simulink model "Third_Order_Polynomial_Clean_Test_Harness"  (R2021b)
settings: Solver=FixedStepDiscrete  StartTime=0.0  StopTime=56  FixedStep=0.001  RelTol=1e-3
libraries: simulink_extras x2
settings Model: Creator=salva  LastModifiedBy=salva
settings DataIOCC: ReturnWorkspaceOutputsName=cubic_out
settings OptimizationCC: DefaultParameterBehavior=Inlined  EnhancedBackFolding=on  PassReuseOutputArgsAs=Individual arguments  ZeroExternalMemoryAtStartup=off  ZeroInternalMemoryAtStartup=off  OptimizeBlockOrder=speed  DifferentSizesBufferReuse=on  OptimizationCustomize=off  EfficientTunableParamExpr=on
settings DebuggingCC: ParameterTunabilityLossMsg=error
settings SFSimCC: MATLABDynamicMemAlloc=off
settings RTWCC: Description=Embedded Coder  SystemTargetFile=ert.tlc  TemplateMakefile=ert_default_tmf
settings CodeAppCC: ForceParamTrailComments=on  IgnoreCustomStorageClasses=off  OperatorAnnotations=on  SimulinkDataObjDesc=on  SFDataObjDesc=on  InsertBlockDesc=on
settings ERTTargetCC: TargetLangStandard=C99 (ISO)  GenerateSampleERTMain=on  InlinedParameterPlacement=NonHierarchical  ERTCustomFileTemplate=example_file_process.tlc

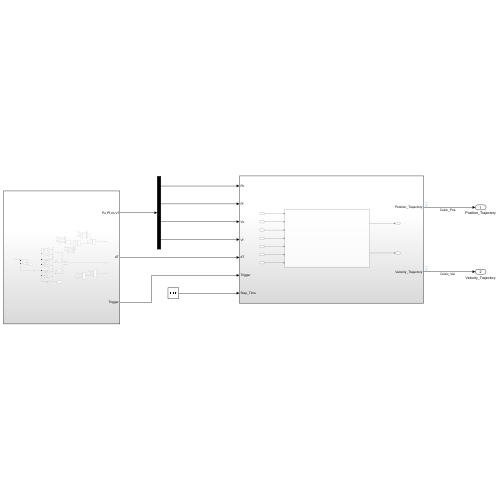
[thumbnail: Simulink's stored preview of the top-level diagram]
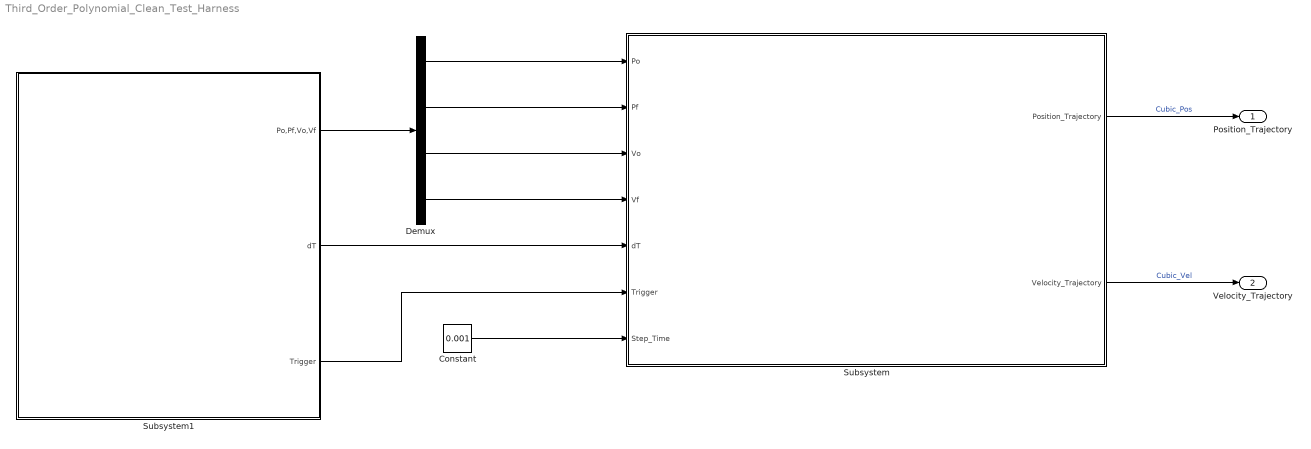
== system Third_Order_Polynomial_Clean_Test_Harness ==
  Constant : Constant  Value=0.001
  Demux : Demux
  Subsystem : Subsystem
  Subsystem1 : Subsystem
  Position_Trajectory : Outport
  Velocity_Trajectory : Outport  Port=2
  wires:
  Demux/1 -> Subsystem/1(Po)
  Demux/2 -> Subsystem/2(Pf)
  Demux/3 -> Subsystem/3(Vo)
  Demux/4 -> Subsystem/4(Vf)
  Subsystem1/2(dT) -> Subsystem/5(dT)
  Subsystem1/3(Trigger) -> Subsystem/6(Trigger)
  Constant/1 -> Subsystem/7(Step_Time)
  Subsystem/1(Position_Trajectory) -> Position_Trajectory/1  "Cubic_Pos"
  Subsystem/2(Velocity_Trajectory) -> Velocity_Trajectory/1  "Cubic_Vel"
  Subsystem1/1(Po,Pf,Vo,Vf) -> Demux/1

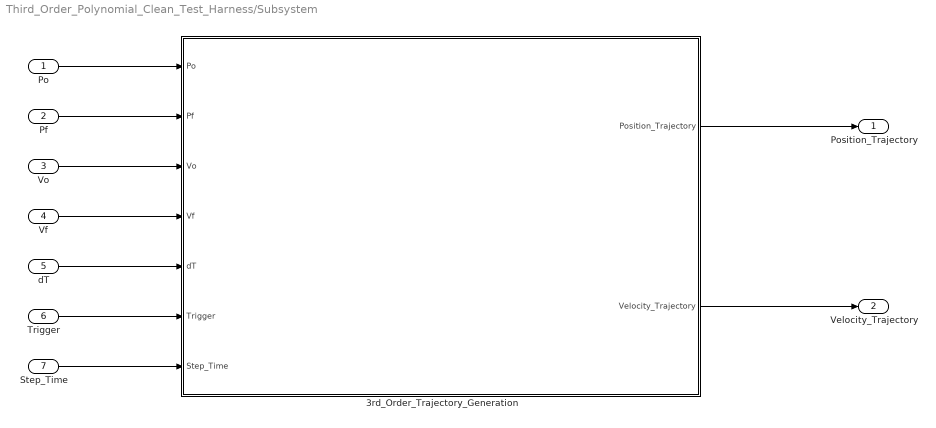
== system Third_Order_Polynomial_Clean_Test_Harness/Subsystem ==
  Po : Inport
  Pf : Inport  Port=2
  Vo : Inport  Port=3
  Vf : Inport  Port=4
  dT : Inport  Port=5
  Trigger : Inport  Port=6
  Step_Time : Inport  Port=7
  3rd_Order_Trajectory_Generation : Subsystem
  Position_Trajectory : Outport
  Velocity_Trajectory : Outport  Port=2
  wires:
  Vf/1 -> 3rd_Order_Trajectory_Generation/4(Vf)
  Trigger/1 -> 3rd_Order_Trajectory_Generation/6(Trigger)
  Pf/1 -> 3rd_Order_Trajectory_Generation/2(Pf)
  3rd_Order_Trajectory_Generation/2(Velocity_Trajectory) -> Velocity_Trajectory/1
  Po/1 -> 3rd_Order_Trajectory_Generation/1(Po)
  3rd_Order_Trajectory_Generation/1(Position_Trajectory) -> Position_Trajectory/1
  dT/1 -> 3rd_Order_Trajectory_Generation/5(dT)
  Vo/1 -> 3rd_Order_Trajectory_Generation/3(Vo)
  Step_Time/1 -> 3rd_Order_Trajectory_Generation/7(Step_Time)

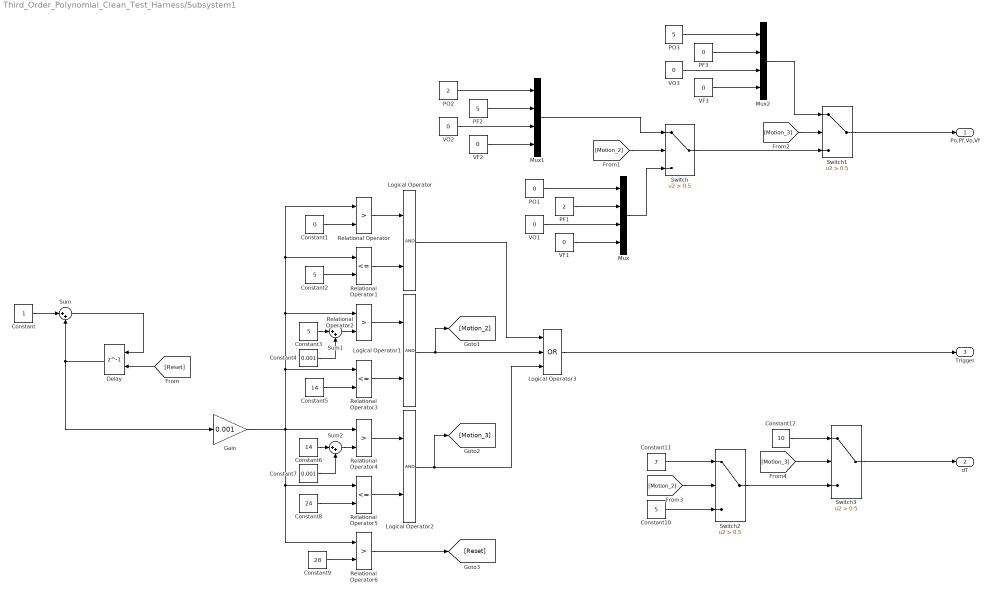
== system Third_Order_Polynomial_Clean_Test_Harness/Subsystem1 ==
  Constant : Constant
  Constant1 : Constant  Value=0
  Constant10 : Constant  Value=5
  Constant11 : Constant  Value=7
  Constant12 : Constant  Value=10
  Constant2 : Constant  Value=5
  Constant3 : Constant  Value=5
  Constant4 : Constant  Value=0.001
  Constant5 : Constant  Value=14
  Constant6 : Constant  Value=14
  Constant7 : Constant  Value=0.001
  Constant8 : Constant  Value=24
  Constant9 : Constant  Value=28
  Delay : Delay  DelayLength=1  ExternalReset=Rising
      settings: InputPortMap=u0,r5
  Gain : Gain  Gain=0.001
  Logical Operator : Logic  AllPortsSameDT=off  OutDataTypeStr=boolean
  Logical Operator1 : Logic  AllPortsSameDT=off  OutDataTypeStr=boolean
  Logical Operator2 : Logic  AllPortsSameDT=off  OutDataTypeStr=boolean
  Logical Operator3 : Logic  Operator=OR  Inputs=3  AllPortsSameDT=off  OutDataTypeStr=boolean
  Mux : Mux
  Mux1 : Mux
  Mux2 : Mux
  PF1 : Constant  Value=2
  PF2 : Constant  Value=5
  PF3 : Constant  Value=0
  PO1 : Constant  Value=0
  PO2 : Constant  Value=2
  PO3 : Constant  Value=5
  Relational Operator{,2,4,6} (4 alike) : RelationalOperator  Operator=>  OutDataTypeStr=boolean  RndMeth=Simplest
  Relational Operator1 : RelationalOperator  Operator=<=  OutDataTypeStr=boolean  RndMeth=Simplest
  Relational Operator3 : RelationalOperator  Operator=<=  OutDataTypeStr=boolean  RndMeth=Simplest
  Relational Operator5 : RelationalOperator  Operator=<=  OutDataTypeStr=boolean  RndMeth=Simplest
  Sum : Sum  Inputs=|++
  Sum1 : Sum  Inputs=|++
  Sum2 : Sum  Inputs=|++
  Switch{,1..3} (4 alike) : Switch  Criteria=u2 > Threshold  Threshold=0.5
  VF1 : Constant  Value=0
  VF2 : Constant  Value=0
  VF3 : Constant  Value=0
  VO1 : Constant  Value=0
  VO2 : Constant  Value=0
  VO3 : Constant  Value=0
  Po,Pf,Vo,Vf : Outport
  dT : Outport  Port=2
  Trigger : Outport  Port=3
  wires:
  VF2/1 -> Mux1/4
  Delay/1 -> Sum/2, Gain/1
  Sum1/1 -> Relational Operator2/2
  Constant3/1 -> Sum1/1
  Constant1/1 -> Relational Operator/2
  VO2/1 -> Mux1/3
  Gain/1 -> Relational Operator/1, Relational Operator1/1, Relational Operator2/1, Relational Operator3/1, Relational Operator6/1, Relational Operator5/1, Relational Operator4/1
  Switch1/1 -> Po,Pf,Vo,Vf/1
  Relational Operator3/1 -> Logical Operator1/2
  Switch/1 -> Switch1/3
  Constant/1 -> Sum/1
  Logical Operator2/1 -> [Motion_3], Logical Operator3/3
  Sum2/1 -> Relational Operator4/2
  PO1/1 -> Mux/1
  [Motion_2] -> Switch/2
  VF1/1 -> Mux/4
  Constant6/1 -> Sum2/1
  Constant8/1 -> Relational Operator5/2
  Constant7/1 -> Sum2/2
  Constant9/1 -> Relational Operator6/2
  Relational Operator1/1 -> Logical Operator/2
  PO3/1 -> Mux2/1
  Relational Operator/1 -> Logical Operator/1
  Relational Operator5/1 -> Logical Operator2/2
  [Reset] -> Delay/2
  Mux2/1 -> Switch1/1
  Relational Operator4/1 -> Logical Operator2/1
  Sum/1 -> Delay/1
  Mux1/1 -> Switch/1
  PF3/1 -> Mux2/2
  Constant4/1 -> Sum1/2
  VF3/1 -> Mux2/4
  Logical Operator1/1 -> [Motion_2], Logical Operator3/2
  [Motion_3] -> Switch1/2
  Constant2/1 -> Relational Operator1/2
  VO3/1 -> Mux2/3
  Logical Operator3/1 -> Trigger/1
  Logical Operator/1 -> Logical Operator3/1
  Constant5/1 -> Relational Operator3/2
  Mux/1 -> Switch/3
  PF2/1 -> Mux1/2
  PO2/1 -> Mux1/1
  Relational Operator2/1 -> Logical Operator1/1
  Relational Operator6/1 -> [Reset]
  PF1/1 -> Mux/2
  VO1/1 -> Mux/3
  [Motion_2] -> Switch2/2
  Switch2/1 -> Switch3/3
  [Motion_3] -> Switch3/2
  Constant10/1 -> Switch2/3
  Constant11/1 -> Switch2/1
  Constant12/1 -> Switch3/1
  Switch3/1 -> dT/1

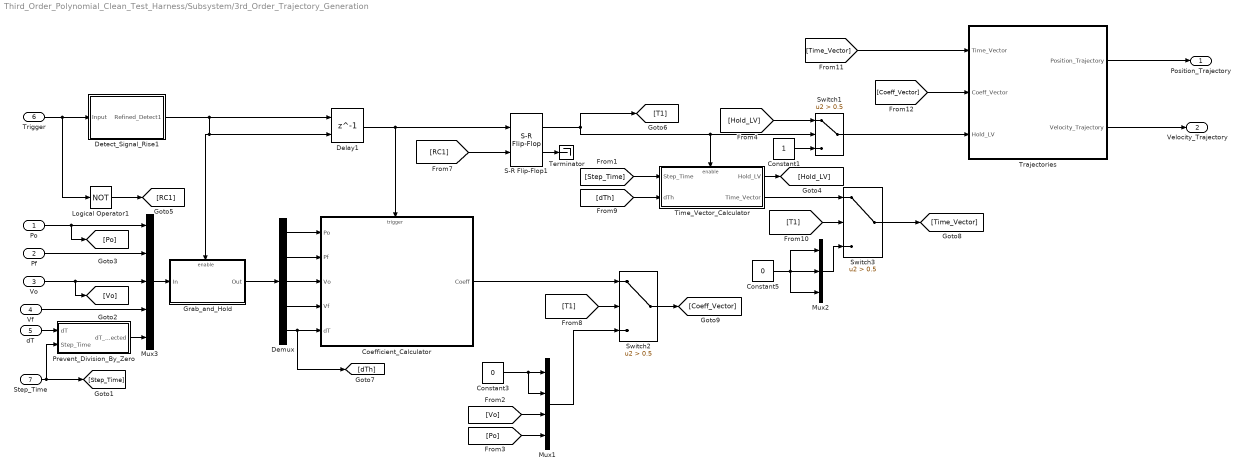
== system Third_Order_Polynomial_Clean_Test_Harness/Subsystem/3rd_Order_Trajectory_Generation ==
  Po : Inport
  Pf : Inport  Port=2
  Vo : Inport  Port=3
  Vf : Inport  Port=4
  dT : Inport  Port=5
  Trigger : Inport  Port=6
  Step_Time : Inport  Port=7
  Coefficient_Calculator : Subsystem
  Constant1 : Constant
  Constant3 : Constant  Value=0
  Constant5 : Constant  Value=0
  Delay1 : Delay  DelayLength=1  InitialConditionSource=Input port
      settings: InputPortMap=u0,p4
  Demux : Demux  Outputs=5
  Detect_Signal_Rise1 : Subsystem
  Grab_and_Hold : Subsystem
  Logical Operator1 : Logic  Operator=NOT  AllPortsSameDT=off  OutDataTypeStr=boolean
  Mux1 : Mux
  Mux2 : Mux  Inputs=3
  Mux3 : Mux  Inputs=5
  Prevent_Division_By_Zero : Subsystem
  S-R Flip-Flop1 : simulink_extras/Flip Flops/S-R Flip-Flop  initial_condition=0
  Switch1 : Switch  Criteria=u2 > Threshold  Threshold=0.5
  Switch2 : Switch  Criteria=u2 > Threshold  Threshold=0.5
  Switch3 : Switch  Criteria=u2 > Threshold  Threshold=0.5
  Terminator : Terminator
  Time_Vector_Calculator : Subsystem
  Trajectories : Subsystem
  Position_Trajectory : Outport
  Velocity_Trajectory : Outport  Port=2
  wires:
  Trajectories/2(Velocity_Trajectory) -> Velocity_Trajectory/1
  Trajectories/1(Position_Trajectory) -> Position_Trajectory/1
  [Coeff_Vector] -> Trajectories/2(Coeff_Vector)
  [Time_Vector] -> Trajectories/1(Time_Vector)
  Switch2/1 -> [Coeff_Vector]
  Switch3/1 -> [Time_Vector]
  Constant5/1 -> Mux2/2, Mux2/3, Mux2/1
  Mux2/1 -> Switch3/3
  Time_Vector_Calculator/2(Time_Vector) -> Switch3/1
  [T1] -> Switch3/2
  [dTh] -> Time_Vector_Calculator/2(dTh)
  [Step_Time] -> Time_Vector_Calculator/1(Step_Time)
  Coefficient_Calculator/1(Coeff) -> Switch2/1
  [T1] -> Switch2/2
  Mux1/1 -> Switch2/3
  Constant3/1 -> Mux1/2, Mux1/1
  S-R Flip-Flop1/1 -> Time_Vector_Calculator/Enable, Switch1/2, [T1]
  S-R Flip-Flop1/2 -> Terminator/1
  [RC1] -> S-R Flip-Flop1/2
  Logical Operator1/1 -> [RC1]
  Delay1/1 -> Coefficient_Calculator/Trigger, S-R Flip-Flop1/1
  Grab_and_Hold/1(Out) -> Demux/1
  Mux3/1 -> Grab_and_Hold/1(In)
  Detect_Signal_Rise1/1(Refined_Detect1) -> Grab_and_Hold/Enable, Delay1/2, Delay1/1
  Trigger/1 -> Logical Operator1/1, Detect_Signal_Rise1/1(Input)
  dT/1 -> Prevent_Division_By_Zero/1(dT)
  Vo/1 -> [Vo], Mux3/3
  Po/1 -> [Po], Mux3/1
  Step_Time/1 -> Prevent_Division_By_Zero/2(Step_Time), [Step_Time]
  Pf/1 -> Mux3/2
  Vf/1 -> Mux3/4
  Demux/1 -> Coefficient_Calculator/1(Po)
  Demux/2 -> Coefficient_Calculator/2(Pf)
  Demux/3 -> Coefficient_Calculator/3(Vo)
  Demux/4 -> Coefficient_Calculator/4(Vf)
  Demux/5 -> Coefficient_Calculator/5(dT), [dTh]
  Prevent_Division_By_Zero/1(dT_Protected) -> Mux3/5
  [Vo] -> Mux1/3
  [Po] -> Mux1/4
  Constant1/1 -> Switch1/3
  Switch1/1 -> Trajectories/3(Hold_LV)
  Time_Vector_Calculator/1(Hold_LV) -> [Hold_LV]
  [Hold_LV] -> Switch1/1

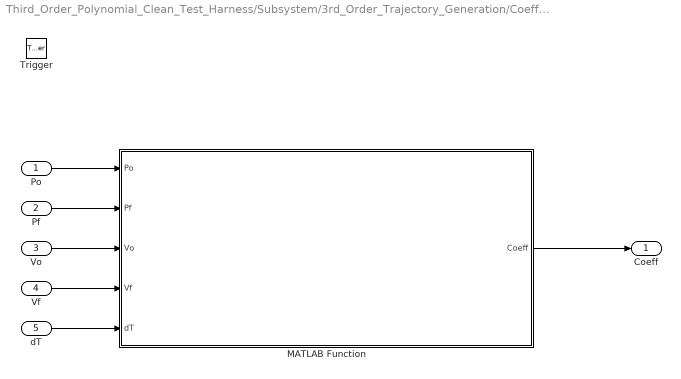
== system Third_Order_Polynomial_Clean_Test_Harness/Subsystem/3rd_Order_Trajectory_Generation/Coefficient_Calculator ==
  Po : Inport
  Pf : Inport  Port=2
  Vo : Inport  Port=3
  Vf : Inport  Port=4
  dT : Inport  Port=5
  Trigger : TriggerPort  VariantControl=(inherit)
  MATLAB Function : MATLAB Function  TreatAsAtomicUnit=on
  Coeff : Outport
  wires:
  MATLAB Function/1(Coeff) -> Coeff/1
  Pf/1 -> MATLAB Function/2(Pf)
  Vf/1 -> MATLAB Function/4(Vf)
  Vo/1 -> MATLAB Function/3(Vo)
  Po/1 -> MATLAB Function/1(Po)
  dT/1 -> MATLAB Function/5(dT)

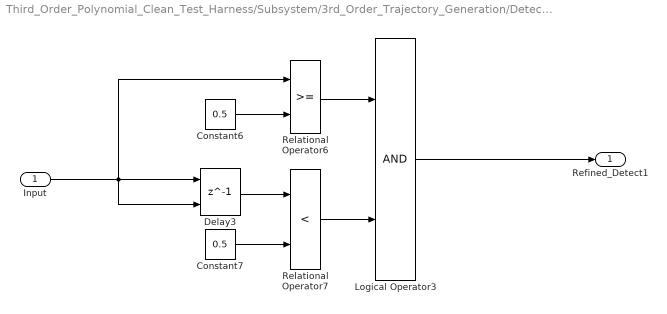
== system Third_Order_Polynomial_Clean_Test_Harness/Subsystem/3rd_Order_Trajectory_Generation/Detect_Signal_Rise1 ==
  Input : Inport
  Constant6 : Constant  Value=0.5
  Constant7 : Constant  Value=0.5
  Delay3 : Delay  DelayLength=1  InitialConditionSource=Input port
      settings: InputPortMap=u0,p4
  Logical Operator3 : Logic  AllPortsSameDT=off  OutDataTypeStr=boolean
  Relational Operator6 : RelationalOperator  OutDataTypeStr=boolean  RndMeth=Simplest
  Relational Operator7 : RelationalOperator  Operator=<  OutDataTypeStr=boolean  RndMeth=Simplest
  Refined_Detect1 : Outport
  wires:
  Delay3/1 -> Relational Operator7/1
  Relational Operator7/1 -> Logical Operator3/2
  Relational Operator6/1 -> Logical Operator3/1
  Input/1 -> Delay3/2, Delay3/1, Relational Operator6/1
  Constant7/1 -> Relational Operator7/2
  Constant6/1 -> Relational Operator6/2
  Logical Operator3/1 -> Refined_Detect1/1

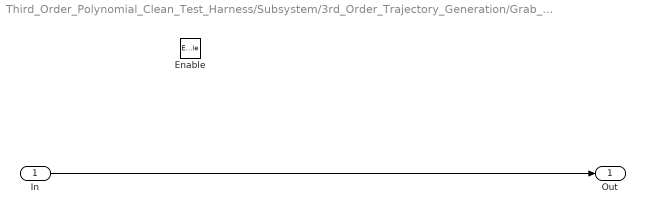
== system Third_Order_Polynomial_Clean_Test_Harness/Subsystem/3rd_Order_Trajectory_Generation/Grab_and_Hold ==
  In : Inport
  Enable : EnablePort  StatesWhenEnabling=reset
  Out : Outport
  wires:
  In/1 -> Out/1

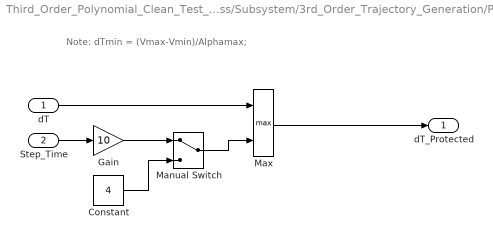
== system Third_Order_Polynomial_Clean_Test_Harness/Subsystem/3rd_Order_Trajectory_Generation/Prevent_Division_By_Zero ==
  note: Note: dTmin = (Vmax-Vmin)/Alphamax;
  dT : Inport
  Step_Time : Inport  Port=2
  Constant : Constant  Value=4
  Gain : Gain  Gain=10
  Manual Switch : ManualSwitch
  Max : MinMax  Function=max  Inputs=2
  dT_Protected : Outport
  wires:
  dT/1 -> Max/1
  Step_Time/1 -> Gain/1
  Gain/1 -> Manual Switch/1
  Max/1 -> dT_Protected/1
  Manual Switch/1 -> Max/2
  Constant/1 -> Manual Switch/2

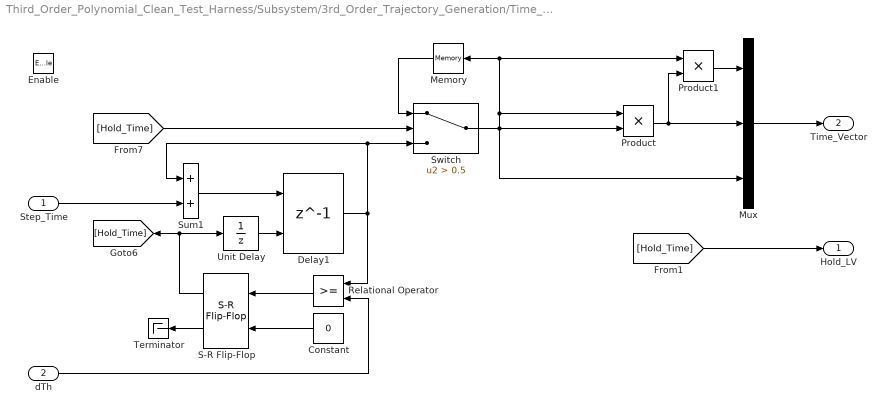
== system Third_Order_Polynomial_Clean_Test_Harness/Subsystem/3rd_Order_Trajectory_Generation/Time_Vector_Calculator ==
  Step_Time : Inport
  dTh : Inport  Port=2
  Enable : EnablePort  StatesWhenEnabling=reset
  Constant : Constant  Value=0  OutDataTypeStr=boolean
  Delay1 : Delay  DelayLength=1  ExternalReset=Level hold
      settings: InputPortMap=u0,r5
  Memory : Memory
  Mux : Mux  Inputs=3
  Product : Product
  Product1 : Product
  Relational Operator : RelationalOperator  OutDataTypeStr=boolean  RndMeth=Simplest
  S-R Flip-Flop : simulink_extras/Flip Flops/S-R Flip-Flop  initial_condition=0
  Sum1 : Sum
  Switch : Switch  Criteria=u2 > Threshold  Threshold=0.5
  Terminator : Terminator
  Unit Delay : UnitDelay  SampleTime=-1  HasFrameUpgradeWarning=on
  Hold_LV : Outport
  Time_Vector : Outport  Port=2
  wires:
  [Hold_Time] -> Hold_LV/1
  Memory/1 -> Switch/1
  Switch/1 -> Product/2, Mux/3, Product/1, Memory/1, Product1/1
  [Hold_Time] -> Switch/2
  Unit Delay/1 -> Delay1/2
  S-R Flip-Flop/1 -> [Hold_Time], Unit Delay/1
  S-R Flip-Flop/2 -> Terminator/1
  Constant/1 -> S-R Flip-Flop/2
  Relational Operator/1 -> S-R Flip-Flop/1
  Mux/1 -> Time_Vector/1
  Product1/1 -> Mux/1
  Product/1 -> Mux/2, Product1/2
  dTh/1 -> Relational Operator/2
  Step_Time/1 -> Sum1/2
  Delay1/1 -> Relational Operator/1, Switch/3, Sum1/1
  Sum1/1 -> Delay1/1

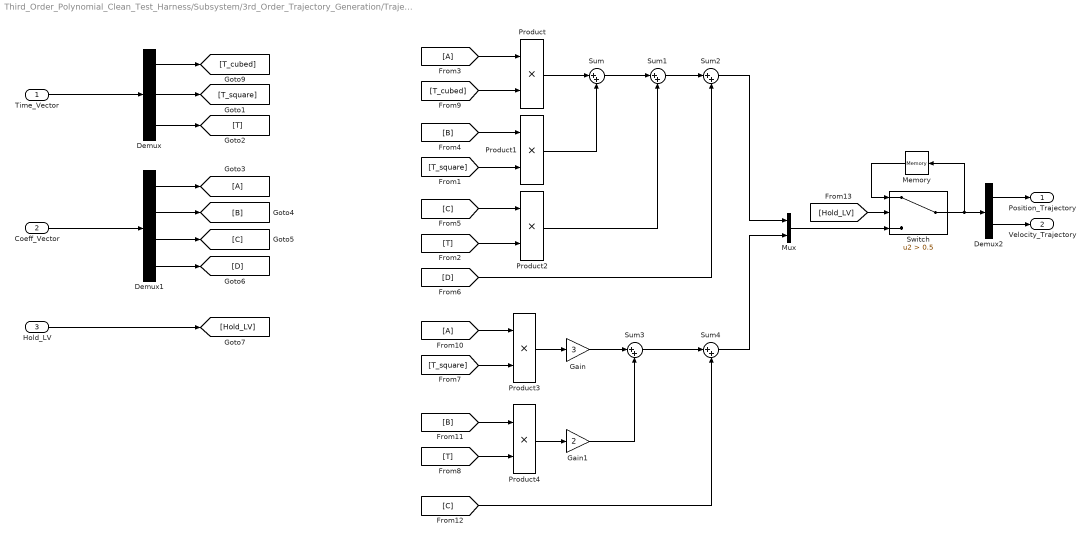
== system Third_Order_Polynomial_Clean_Test_Harness/Subsystem/3rd_Order_Trajectory_Generation/Trajectories ==
  Time_Vector : Inport
  Coeff_Vector : Inport  Port=2
  Hold_LV : Inport  Port=3
  Demux : Demux  Outputs=3
  Demux1 : Demux
  Demux2 : Demux  Outputs=2
  Gain : Gain  Gain=3
  Gain1 : Gain  Gain=2
  Memory : Memory
  Mux : Mux  Inputs=2
  Product{,1..4} (5 alike) : Product
  Sum{,1..4} (5 alike) : Sum  Inputs=|++
  Switch : Switch  Criteria=u2 > Threshold  Threshold=0.5
  Position_Trajectory : Outport
  Velocity_Trajectory : Outport  Port=2
  wires:
  Demux2/2 -> Velocity_Trajectory/1
  Demux2/1 -> Position_Trajectory/1
  [Hold_LV] -> Switch/2
  Memory/1 -> Switch/1
  Switch/1 -> Memory/1, Demux2/1
  Hold_LV/1 -> [Hold_LV]
  Mux/1 -> Switch/3
  Sum4/1 -> Mux/2
  Sum2/1 -> Mux/1
  [C] -> Sum4/2
  Sum3/1 -> Sum4/1
  Gain1/1 -> Sum3/2
  Gain/1 -> Sum3/1
  Product4/1 -> Gain1/1
  [B] -> Product4/1
  [T] -> Product4/2
  Product3/1 -> Gain/1
  [T_square] -> Product3/2
  [A] -> Product3/1
  [D] -> Sum2/2
  Sum1/1 -> Sum2/1
  Product2/1 -> Sum1/2
  [T] -> Product2/2
  [C] -> Product2/1
  Sum/1 -> Sum1/1
  Product1/1 -> Sum/2
  [T_square] -> Product1/2
  [B] -> Product1/1
  Product/1 -> Sum/1
  [T_cubed] -> Product/2
  [A] -> Product/1
  Demux1/4 -> [D]
  Demux1/3 -> [C]
  Demux1/2 -> [B]
  Demux1/1 -> [A]
  Demux/3 -> [T]
  Demux/1 -> [T_cubed]
  Demux/2 -> [T_square]
  Coeff_Vector/1 -> Demux1/1
  Time_Vector/1 -> Demux/1

== matlab function Third_Order_Polynomial_Clean_Test_Harness/Subsystem/3rd_Order_Trajectory_Generation/Coefficient_Calculator/MATLAB Function ==
  data: Po input; Coeff output; Pf input; Vo input; Vf input; dT input
function Coeff = solve_cubic(Po, Pf, Vo, Vf, dT)

% Position = (A)*dT^3 + (B)*dT^2 + (C)*dT + D
% Velocity = (3A)*dT^2 + (2B)*dT + C
% Where P(t=0) = Po; P(t=dT) = Pf; V(t=0)=Vo; V(t=dT) = Vf

% Calculate dT multiplication to reduce math loading
dT2 = dT*dT;
dT3 = dT2*dT;

% Calculate Coefficients
D = Po;
C = Vo;
B = (-((Vf+2*C)*dT)+3*(Pf-D))/(dT2);
A = ((Vf+C)*dT-(2*(Pf-D)))/(dT3);

% Output Coefficients
Coeff = [A,B,C,D];
